simulink model "lqg"  (R2018b)
settings: Solver=VariableStepAuto  StartTime=0.0  StopTime=10.0  RelTol=1e-3
values from neighbouring files (symbols this model uses):
  A = a    [rscale.m]
  B = b    [rscale.m]
  C = c    [rscale.m]
undefined symbols (not defined in the file or in its folder): G, kalmf, L
libraries: simulink x2
settings Model: Creator=adelina  LastModifiedBy=adelina

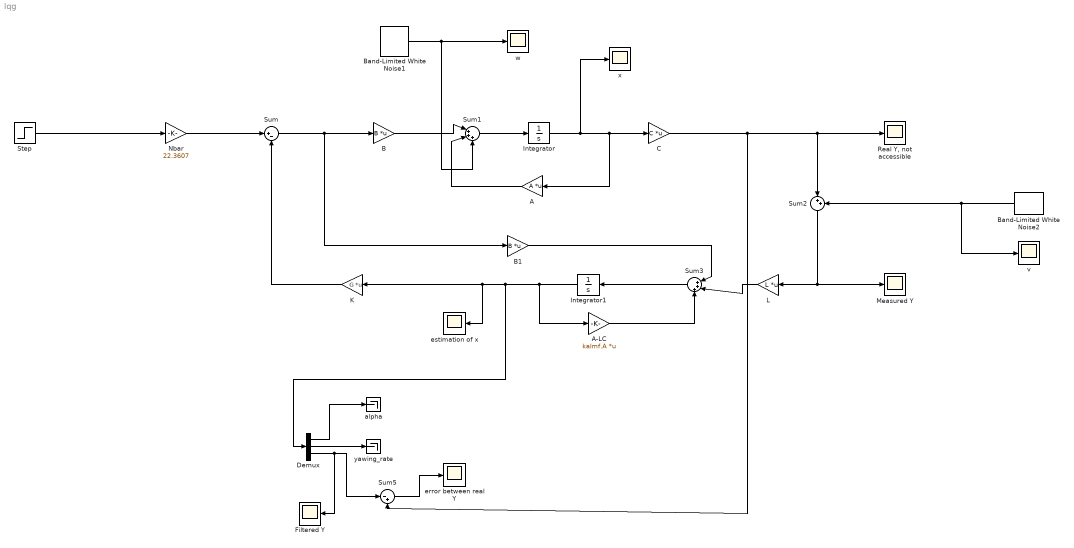
== system lqg ==
  A : Gain  Gain=A  Multiplication=Matrix(K*u)
  A-LC : Gain  Gain=kalmf.A  Multiplication=Matrix(K*u)
  B : Gain  Gain=B  Multiplication=Matrix(K*u)
  B1 : Gain  Gain=B  Multiplication=Matrix(K*u)
  Band-Limited White Noise1 : simulink/Sources/Band-Limited White Noise  Cov=[0.0000004]  Ts=0.01  seed=[23]
  Band-Limited White Noise2 : simulink/Sources/Band-Limited White Noise  Cov=[0.000001]  Ts=0.01  seed=[23]
  C : Gain  Gain=C  Multiplication=Matrix(K*u)
  Demux : Demux  Outputs=3
  Filtered Y : Scope
  Integrator : Integrator
  Integrator1 : Integrator
  K : Gain  Gain=G  Multiplication=Matrix(K*u) (u vector)
  L : Gain  Gain=L  Multiplication=Matrix(K*u)
  Measured Y : Scope
  Nbar : Gain  Gain=22.3607
  "Real Y, not accessible" : Scope
  Step : Step  After=0.2  SampleTime=0
  Sum : Sum  Inputs=|+-
  Sum1 : Sum  Inputs=|+++
  Sum2 : Sum  Inputs=|++
  Sum3 : Sum  Inputs=|+++
  Sum5 : Sum  Inputs=|-+
  alpha : Terminator
  error between real Y : Scope
  estimation of x : Scope
  v : Scope
  w : Scope
  "x " : Scope
  yawing_rate : Terminator
  wires:
  Step/1 -> Nbar/1
  Nbar/1 -> Sum/1
  Sum/1 -> B/1, B1/1
  B/1 -> Sum1/1
  Sum1/1 -> Integrator/1
  Integrator/1 -> "x "/1, C/1, A/1
  C/1 -> Sum2/1, "Real Y, not accessible"/1, Sum5/2
  A/1 -> Sum1/2
  Sum2/1 -> Measured Y/1, L/1
  L/1 -> Sum3/2
  B1/1 -> Sum3/1
  Sum3/1 -> Integrator1/1
  Integrator1/1 -> A-LC/1, Demux/1, estimation of x/1, K/1
  A-LC/1 -> Sum3/3
  Band-Limited White Noise2/1 -> v/1, Sum2/2
  K/1 -> Sum/2
  Band-Limited White Noise1/1 -> Sum1/3, w/1
  Demux/1 -> alpha/1
  Demux/3 -> Filtered Y/1, Sum5/1
  Demux/2 -> yawing_rate/1
  Sum5/1 -> error between real Y/1
